simulink model "parrot_motor_speed"  (R2022a)
settings: Solver=FixedStepAuto  StartTime=0.0  StopTime=100  RelTol=1e-3  EnableMultiTasking=on
InitFcn:
  | load('BusDefinitions.mat')
undefined symbols (not defined in the file): codertarget, Ts
libraries: simulink x34
settings Model: SimulationMode=external  ExtModeTrigDuration=80  Creator=The MathWorks, Inc.  LastModifiedBy=Muhammad Ahmad Basra
settings SolverCC: AlgebraicLoopSolver=TrustRegion  PositivePriorityOrder=on
settings DataIOCC: ReturnWorkspaceOutputs=off
settings OptimizationCC: PassReuseOutputArgsThreshold=0  MaxStackSize=64
settings DebuggingCC: ParameterOverflowMsg=none  ParameterPrecisionLossMsg=none  ParameterTunabilityLossMsg=error  UnconnectedInputMsg=warning  UnconnectedOutputMsg=warning  UnconnectedLineMsg=warning  PregeneratedLibrarySubsystemCodeDiagnostic=none  SFMachineParentedDataDiag=warning  ArithmeticOperatorsInVariantConditions=warning
settings HardwareCC: ProdBitPerPointer=32  ProdBitPerSizeT=32  ProdBitPerPtrDiffT=32  ProdLargestAtomicInteger=Long  ProdWordSize=32  ProdHWDeviceType=ARM Compatible->ARM 9  UseEmbeddedCoderFeatures=off  UseSimulinkCoderFeatures=off
settings SFSimCC: SimUseLocalCustomCode=off  MATLABDynamicMemAlloc=off  CustomCodeUndefinedFunction=UseInterfaceOnly
settings RTWCC: SystemTargetFile=ert.tlc  HardwareBoard=PARROT Mambo  TemplateMakefile=ert_default_tmf  GenerateReport=on  RTWUseLocalCustomCode=off  Toolchain=Sourcery G++ Lite GNU Toolchain for Drones  LaunchReport=on
settings CodeAppCC: ForceParamTrailComments=on  OperatorAnnotations=on  StateflowObjectComments=on
settings ERTTargetCC: ERTCustomFileBanners=off  SupportContinuousTime=on  SupportNonInlinedSFcns=on  RemoveResetFunc=off  ModelStepFunctionPrototypeControlCompliant=off

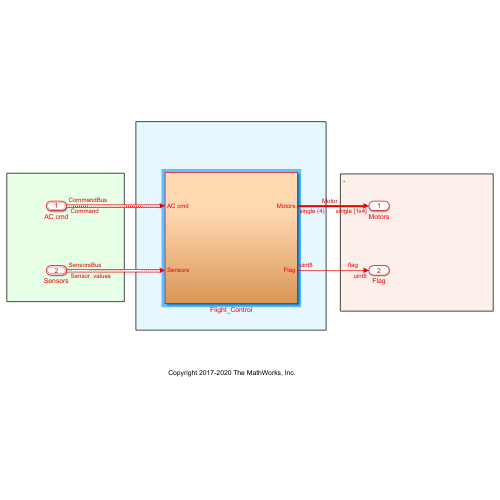
[thumbnail: Simulink's stored preview of the top-level diagram]
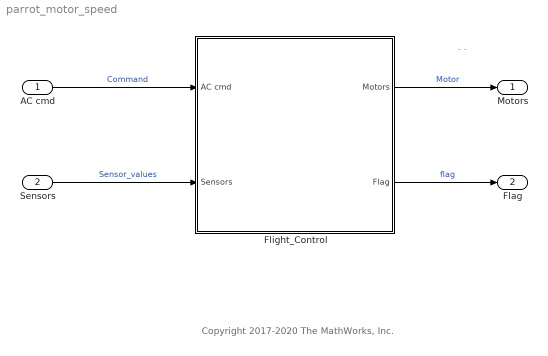
== system parrot_motor_speed ==
  note: .
      |
      |
      | .
  note: Copyright 2017-2020 The MathWorks, Inc.
  AC cmd : Inport  OutDataTypeStr=Bus: CommandBus  BusOutputAsStruct=on
  Sensors : Inport  Port=2  OutDataTypeStr=Bus: SensorsBus  BusOutputAsStruct=on
  Flight_Control : Subsystem  InitFcn=codertarget.parrot.internal.fcsSubsystemCallback(gcb);
  Motors : Outport  OutDataTypeStr=single  PortDimensions=[1 4]  VectorParamsAs1DForOutWhenUnconnected=off
  Flag : Outport  Port=2  OutDataTypeStr=uint8  PortDimensions=1  VectorParamsAs1DForOutWhenUnconnected=off
  wires:
  Flight_Control/1(Motors) -> Motors/1  "Motor"
  AC cmd/1 -> Flight_Control/1(AC cmd)  "Command"
  Sensors/1 -> Flight_Control/2(Sensors)  "Sensor_values"
  Flight_Control/2(Flag) -> Flag/1  "flag"

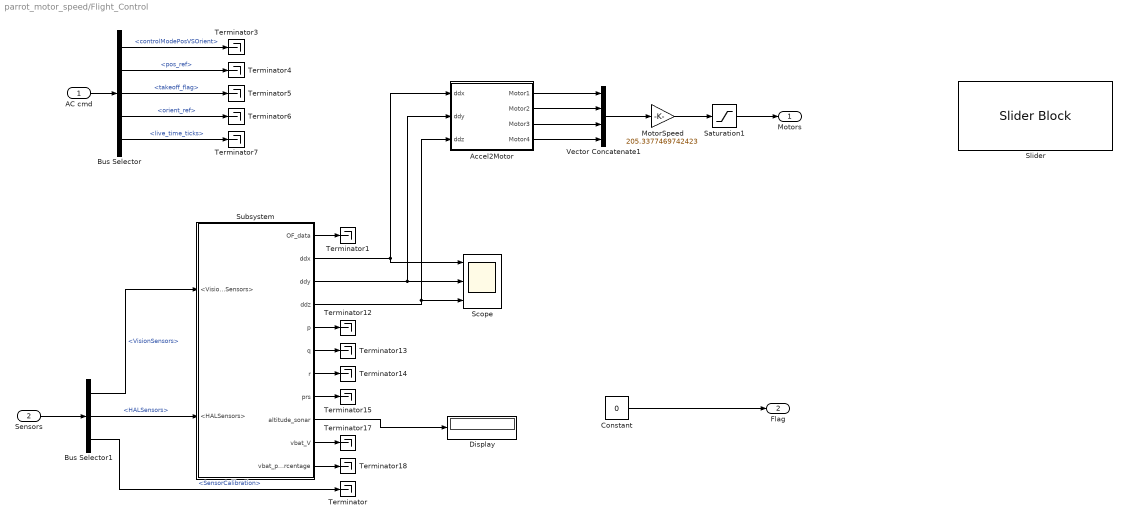
== system parrot_motor_speed/Flight_Control ==
  AC cmd : Inport
  Sensors : Inport  Port=2
  Accel2Motor : Subsystem
  Bus Selector : BusSelector  OutputSignals=controlModePosVSOrient,pos_ref,takeoff_flag,orient_ref,live_time_ticks
  Bus Selector1 : BusSelector  OutputSignals=VisionSensors,HALSensors,SensorCalibration
  Constant : Constant  Value=0  OutDataTypeStr=uint8  SampleTime=Ts
  Display : Display
  MotorSpeed : Gain  Gain=205.3377469742423  OutDataTypeStr=single
  Saturation1 : Saturate  UpperLimit=500  LowerLimit=0  OutDataTypeStr=single
  Scope : Scope  NumInputPorts=3
  Slider : SliderBlock  ScaleMax=500
  Subsystem : Subsystem
  Terminator{,1,3..7,12..15,17..18} (13 alike) : Terminator
  Vector Concatenate1 : Concatenate  NumInputs=4
  Motors : Outport  VectorParamsAs1DForOutWhenUnconnected=off
  Flag : Outport  Port=2  VectorParamsAs1DForOutWhenUnconnected=off
  wires:
  AC cmd/1 -> Bus Selector/1
  Sensors/1 -> Bus Selector1/1
  Bus Selector/1 -> Terminator3/1  "<controlModePosVSOrient>"
  Bus Selector/2 -> Terminator4/1  "<pos_ref>"
  Bus Selector/3 -> Terminator5/1  "<takeoff_flag>"
  Bus Selector/4 -> Terminator6/1  "<orient_ref>"
  Bus Selector/5 -> Terminator7/1  "<live_time_ticks>"
  Constant/1 -> Flag/1
  Vector Concatenate1/1 -> MotorSpeed/1
  Accel2Motor/1(Motor1) -> Vector Concatenate1/1
  Accel2Motor/4(Motor4) -> Vector Concatenate1/4
  Accel2Motor/2(Motor2) -> Vector Concatenate1/2
  Accel2Motor/3(Motor3) -> Vector Concatenate1/3
  Saturation1/1 -> Motors/1
  Bus Selector1/1 -> Subsystem/1(<VisionSensors>)  "<VisionSensors>"
  Bus Selector1/2 -> Subsystem/2(<HALSensors>)  "<HALSensors>"
  Bus Selector1/3 -> Terminator/1  "<SensorCalibration>"
  Subsystem/1(OF_data) -> Terminator1/1
  Subsystem/2(ddx) -> Accel2Motor/1(ddx), Scope/1
  Subsystem/3(ddy) -> Accel2Motor/2(ddy), Scope/2
  Subsystem/4(ddz) -> Accel2Motor/3(ddz), Scope/3
  Subsystem/5(p) -> Terminator12/1
  Subsystem/7(r) -> Terminator14/1
  Subsystem/8(prs) -> Terminator15/1
  Subsystem/9(altitude_sonar) -> Display/1
  Subsystem/10(vbat_V) -> Terminator17/1
  Subsystem/11(vbat_percentage) -> Terminator18/1
  Subsystem/6(q) -> Terminator13/1
  MotorSpeed/1 -> Saturation1/1

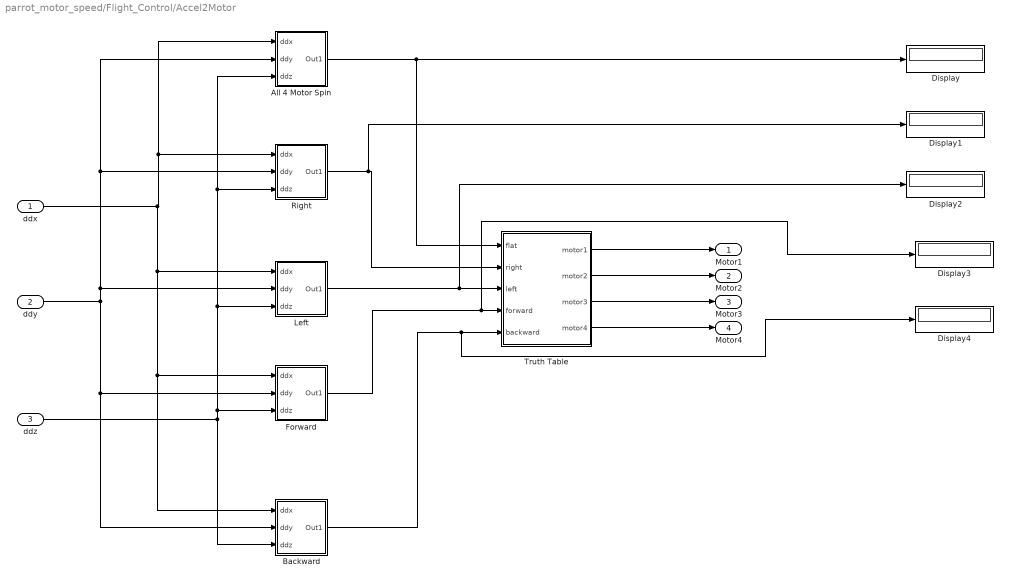
== system parrot_motor_speed/Flight_Control/Accel2Motor ==
  ddx : Inport
  ddy : Inport  Port=2
  ddz : Inport  Port=3
  All 4 Motor Spin : Subsystem
  Backward : Subsystem
  Display{,1..4} (5 alike) : Display
  Forward : Subsystem
  Left : Subsystem
  Right : Subsystem
  Truth Table : Truth Table  TreatAsAtomicUnit=on
  Motor1 : Outport  VectorParamsAs1DForOutWhenUnconnected=off
  Motor2 : Outport  Port=2  VectorParamsAs1DForOutWhenUnconnected=off
  Motor3 : Outport  Port=3  VectorParamsAs1DForOutWhenUnconnected=off
  Motor4 : Outport  Port=4  VectorParamsAs1DForOutWhenUnconnected=off
  wires:
  All 4 Motor Spin/1(Out1) -> Display/1, Truth Table/1(flat)
  Right/1(Out1) -> Display1/1, Truth Table/2(right)
  Left/1(Out1) -> Display2/1, Truth Table/3(left)
  Forward/1(Out1) -> Display3/1, Truth Table/4(forward)
  Backward/1(Out1) -> Display4/1, Truth Table/5(backward)
  Truth Table/1(motor1) -> Motor1/1
  Truth Table/2(motor2) -> Motor2/1
  Truth Table/3(motor3) -> Motor3/1
  Truth Table/4(motor4) -> Motor4/1
  ddx/1 -> Backward/1(ddx), Forward/1(ddx), Left/1(ddx), Right/1(ddx), All 4 Motor Spin/1(ddx)
  ddy/1 -> Left/2(ddy), Right/2(ddy), All 4 Motor Spin/2(ddy), Backward/2(ddy), Forward/2(ddy)
  ddz/1 -> Backward/3(ddz), All 4 Motor Spin/3(ddz), Right/3(ddz), Left/3(ddz), Forward/3(ddz)

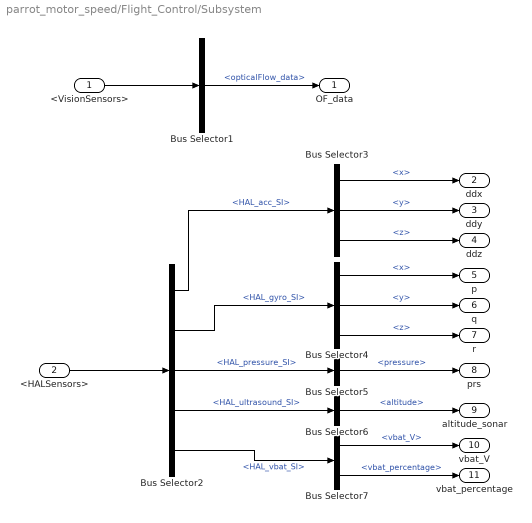
== system parrot_motor_speed/Flight_Control/Subsystem ==
  <VisionSensors> : Inport
  <HALSensors> : Inport  Port=2
  Bus Selector1 : BusSelector  OutputSignals=opticalFlow_data
  Bus Selector2 : BusSelector  OutputSignals=HAL_acc_SI,HAL_gyro_SI,HAL_pressure_SI,HAL_ultrasound_SI,HAL_vbat_SI
  Bus Selector3 : BusSelector  OutputSignals=x,y,z
  Bus Selector4 : BusSelector  OutputSignals=x,y,z
  Bus Selector5 : BusSelector  OutputSignals=pressure
  Bus Selector6 : BusSelector  OutputSignals=altitude
  Bus Selector7 : BusSelector  OutputSignals=vbat_V,vbat_percentage
  OF_data : Outport  VectorParamsAs1DForOutWhenUnconnected=off
  ddx : Outport  Port=2  VectorParamsAs1DForOutWhenUnconnected=off
  ddy : Outport  Port=3  VectorParamsAs1DForOutWhenUnconnected=off
  ddz : Outport  Port=4  VectorParamsAs1DForOutWhenUnconnected=off
  p : Outport  Port=5  VectorParamsAs1DForOutWhenUnconnected=off
  q : Outport  Port=6  VectorParamsAs1DForOutWhenUnconnected=off
  r : Outport  Port=7  VectorParamsAs1DForOutWhenUnconnected=off
  prs : Outport  Port=8  VectorParamsAs1DForOutWhenUnconnected=off
  altitude_sonar : Outport  Port=9  VectorParamsAs1DForOutWhenUnconnected=off
  vbat_V : Outport  Port=10  VectorParamsAs1DForOutWhenUnconnected=off
  vbat_percentage : Outport  Port=11  VectorParamsAs1DForOutWhenUnconnected=off
  wires:
  <VisionSensors>/1 -> Bus Selector1/1
  <HALSensors>/1 -> Bus Selector2/1
  Bus Selector1/1 -> OF_data/1  "<opticalFlow_data>"
  Bus Selector2/1 -> Bus Selector3/1  "<HAL_acc_SI>"
  Bus Selector2/2 -> Bus Selector4/1  "<HAL_gyro_SI>"
  Bus Selector2/3 -> Bus Selector5/1  "<HAL_pressure_SI>"
  Bus Selector2/4 -> Bus Selector6/1  "<HAL_ultrasound_SI>"
  Bus Selector2/5 -> Bus Selector7/1  "<HAL_vbat_SI>"
  Bus Selector3/1 -> ddx/1  "<x>"
  Bus Selector3/2 -> ddy/1  "<y>"
  Bus Selector3/3 -> ddz/1  "<z>"
  Bus Selector4/2 -> q/1  "<y>"
  Bus Selector4/1 -> p/1  "<x>"
  Bus Selector4/3 -> r/1  "<z>"
  Bus Selector5/1 -> prs/1  "<pressure>"
  Bus Selector6/1 -> altitude_sonar/1  "<altitude>"
  Bus Selector7/1 -> vbat_V/1  "<vbat_V>"
  Bus Selector7/2 -> vbat_percentage/1  "<vbat_percentage>"

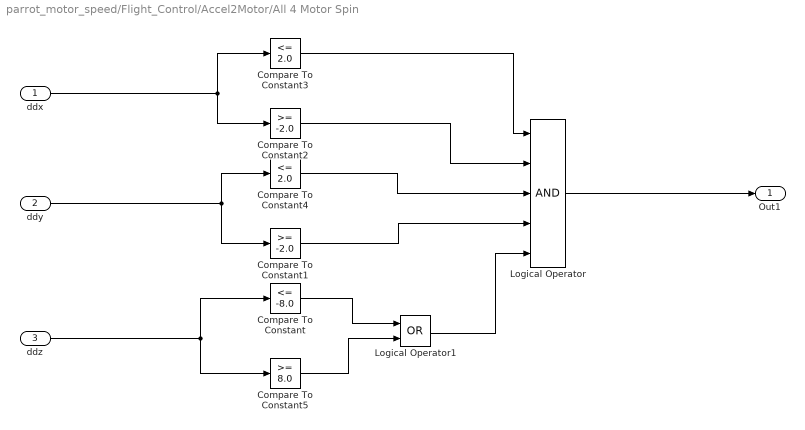
== system parrot_motor_speed/Flight_Control/Accel2Motor/All 4 Motor Spin ==
  ddx : Inport
  ddy : Inport  Port=2
  ddz : Inport  Port=3
  Compare To Constant : simulink/Logic and Bit Operations/Compare To Constant  relop=<=  const=-8.0  OutDataTypeStr=boolean
  Compare To Constant1 : simulink/Logic and Bit Operations/Compare To Constant  relop=>=  const=-2.0  OutDataTypeStr=boolean
  Compare To Constant2 : simulink/Logic and Bit Operations/Compare To Constant  relop=>=  const=-2.0  OutDataTypeStr=boolean
  Compare To Constant3 : simulink/Logic and Bit Operations/Compare To Constant  relop=<=  const=2.0  OutDataTypeStr=boolean
  Compare To Constant4 : simulink/Logic and Bit Operations/Compare To Constant  relop=<=  const=2.0  OutDataTypeStr=boolean
  Compare To Constant5 : simulink/Logic and Bit Operations/Compare To Constant  relop=>=  const=8.0  OutDataTypeStr=boolean
  Logical Operator : Logic  Inputs=5  AllPortsSameDT=off  OutDataTypeStr=boolean
  Logical Operator1 : Logic  Operator=OR  AllPortsSameDT=off  OutDataTypeStr=boolean
  Out1 : Outport  VectorParamsAs1DForOutWhenUnconnected=off
  wires:
  Compare To Constant4/1 -> Logical Operator/3
  ddy/1 -> Compare To Constant1/1, Compare To Constant4/1
  ddz/1 -> Compare To Constant5/1, Compare To Constant/1
  Compare To Constant/1 -> Logical Operator1/1
  ddx/1 -> Compare To Constant3/1, Compare To Constant2/1
  Compare To Constant1/1 -> Logical Operator/4
  Compare To Constant3/1 -> Logical Operator/1
  Logical Operator1/1 -> Logical Operator/5
  Compare To Constant5/1 -> Logical Operator1/2
  Compare To Constant2/1 -> Logical Operator/2
  Logical Operator/1 -> Out1/1

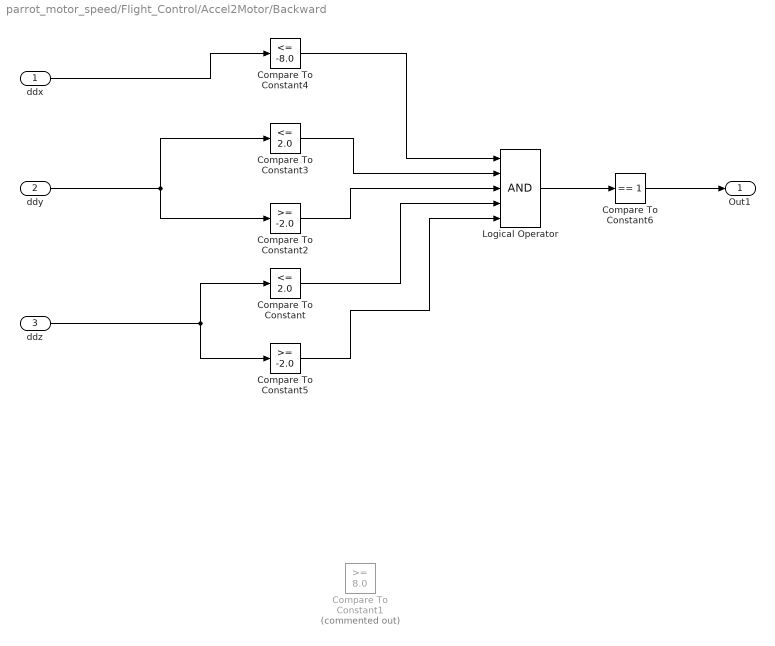
== system parrot_motor_speed/Flight_Control/Accel2Motor/Backward ==
  ddx : Inport
  ddy : Inport  Port=2
  ddz : Inport  Port=3
  Compare To Constant : simulink/Logic and Bit Operations/Compare To Constant  relop=<=  const=2.0  OutDataTypeStr=boolean
  Compare To Constant1 : simulink/Logic and Bit Operations/Compare To Constant  Commented=on  relop=>=  const=8.0  OutDataTypeStr=boolean
  Compare To Constant2 : simulink/Logic and Bit Operations/Compare To Constant  relop=>=  const=-2.0  OutDataTypeStr=boolean
  Compare To Constant3 : simulink/Logic and Bit Operations/Compare To Constant  relop=<=  const=2.0  OutDataTypeStr=boolean
  Compare To Constant4 : simulink/Logic and Bit Operations/Compare To Constant  relop=<=  const=-8.0  OutDataTypeStr=boolean
  Compare To Constant5 : simulink/Logic and Bit Operations/Compare To Constant  relop=>=  const=-2.0  OutDataTypeStr=boolean
  Compare To Constant6 : simulink/Logic and Bit Operations/Compare To Constant  relop===  const=1  OutDataTypeStr=boolean
  Logical Operator : Logic  Inputs=5  AllPortsSameDT=off  OutDataTypeStr=boolean
  Out1 : Outport  VectorParamsAs1DForOutWhenUnconnected=off
  wires:
  Compare To Constant2/1 -> Logical Operator/3
  Compare To Constant3/1 -> Logical Operator/2
  Compare To Constant4/1 -> Logical Operator/1
  ddx/1 -> Compare To Constant4/1
  ddy/1 -> Compare To Constant2/1, Compare To Constant3/1
  Compare To Constant6/1 -> Out1/1
  Logical Operator/1 -> Compare To Constant6/1
  Compare To Constant5/1 -> Logical Operator/5
  Compare To Constant/1 -> Logical Operator/4
  ddz/1 -> Compare To Constant5/1, Compare To Constant/1

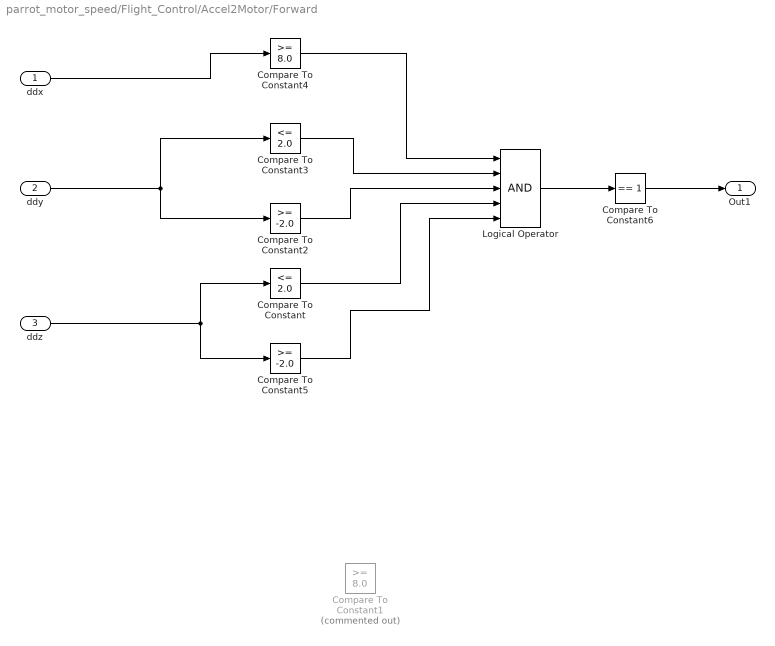
== system parrot_motor_speed/Flight_Control/Accel2Motor/Forward ==
  ddx : Inport
  ddy : Inport  Port=2
  ddz : Inport  Port=3
  Compare To Constant : simulink/Logic and Bit Operations/Compare To Constant  relop=<=  const=2.0  OutDataTypeStr=boolean
  Compare To Constant1 : simulink/Logic and Bit Operations/Compare To Constant  Commented=on  relop=>=  const=8.0  OutDataTypeStr=boolean
  Compare To Constant2 : simulink/Logic and Bit Operations/Compare To Constant  relop=>=  const=-2.0  OutDataTypeStr=boolean
  Compare To Constant3 : simulink/Logic and Bit Operations/Compare To Constant  relop=<=  const=2.0  OutDataTypeStr=boolean
  Compare To Constant4 : simulink/Logic and Bit Operations/Compare To Constant  relop=>=  const=8.0  OutDataTypeStr=boolean
  Compare To Constant5 : simulink/Logic and Bit Operations/Compare To Constant  relop=>=  const=-2.0  OutDataTypeStr=boolean
  Compare To Constant6 : simulink/Logic and Bit Operations/Compare To Constant  relop===  const=1  OutDataTypeStr=boolean
  Logical Operator : Logic  Inputs=5  AllPortsSameDT=off  OutDataTypeStr=boolean
  Out1 : Outport  VectorParamsAs1DForOutWhenUnconnected=off
  wires:
  ddz/1 -> Compare To Constant/1, Compare To Constant5/1
  Compare To Constant/1 -> Logical Operator/4
  Compare To Constant5/1 -> Logical Operator/5
  Logical Operator/1 -> Compare To Constant6/1
  Compare To Constant6/1 -> Out1/1
  ddy/1 -> Compare To Constant3/1, Compare To Constant2/1
  ddx/1 -> Compare To Constant4/1
  Compare To Constant4/1 -> Logical Operator/1
  Compare To Constant3/1 -> Logical Operator/2
  Compare To Constant2/1 -> Logical Operator/3

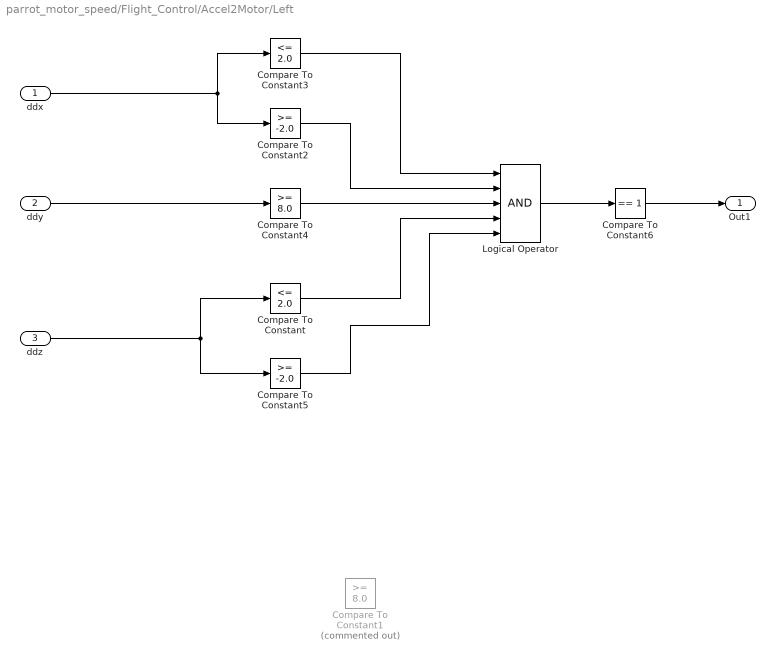
== system parrot_motor_speed/Flight_Control/Accel2Motor/Left ==
  ddx : Inport
  ddy : Inport  Port=2
  ddz : Inport  Port=3
  Compare To Constant : simulink/Logic and Bit Operations/Compare To Constant  relop=<=  const=2.0  OutDataTypeStr=boolean
  Compare To Constant1 : simulink/Logic and Bit Operations/Compare To Constant  Commented=on  relop=>=  const=8.0  OutDataTypeStr=boolean
  Compare To Constant2 : simulink/Logic and Bit Operations/Compare To Constant  relop=>=  const=-2.0  OutDataTypeStr=boolean
  Compare To Constant3 : simulink/Logic and Bit Operations/Compare To Constant  relop=<=  const=2.0  OutDataTypeStr=boolean
  Compare To Constant4 : simulink/Logic and Bit Operations/Compare To Constant  relop=>=  const=8.0  OutDataTypeStr=boolean
  Compare To Constant5 : simulink/Logic and Bit Operations/Compare To Constant  relop=>=  const=-2.0  OutDataTypeStr=boolean
  Compare To Constant6 : simulink/Logic and Bit Operations/Compare To Constant  relop===  const=1  OutDataTypeStr=boolean
  Logical Operator : Logic  Inputs=5  AllPortsSameDT=off  OutDataTypeStr=boolean
  Out1 : Outport  VectorParamsAs1DForOutWhenUnconnected=off
  wires:
  Compare To Constant6/1 -> Out1/1
  Logical Operator/1 -> Compare To Constant6/1
  Compare To Constant5/1 -> Logical Operator/5
  Compare To Constant/1 -> Logical Operator/4
  Compare To Constant4/1 -> Logical Operator/3
  Compare To Constant2/1 -> Logical Operator/2
  Compare To Constant3/1 -> Logical Operator/1
  ddy/1 -> Compare To Constant4/1
  ddz/1 -> Compare To Constant5/1, Compare To Constant/1
  ddx/1 -> Compare To Constant3/1, Compare To Constant2/1

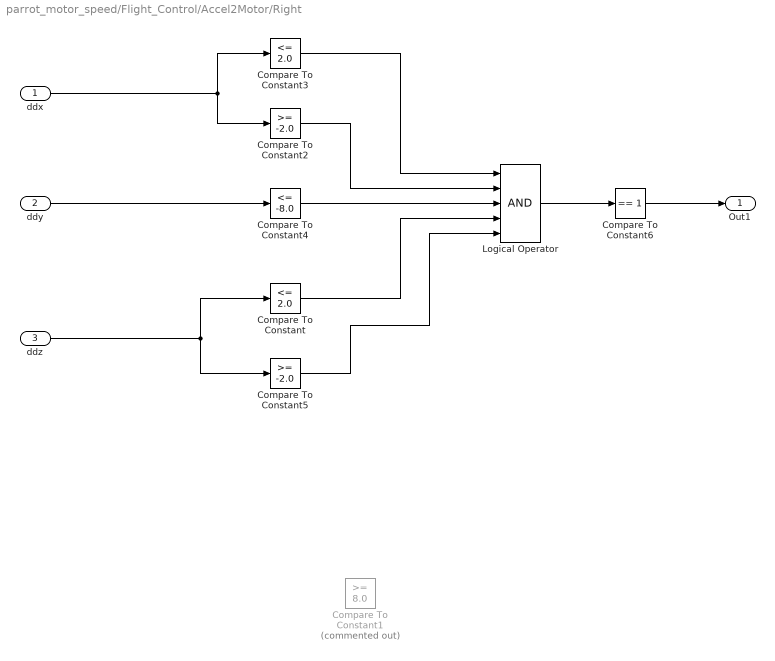
== system parrot_motor_speed/Flight_Control/Accel2Motor/Right ==
  ddx : Inport
  ddy : Inport  Port=2
  ddz : Inport  Port=3
  Compare To Constant : simulink/Logic and Bit Operations/Compare To Constant  relop=<=  const=2.0  OutDataTypeStr=boolean
  Compare To Constant1 : simulink/Logic and Bit Operations/Compare To Constant  Commented=on  relop=>=  const=8.0  OutDataTypeStr=boolean
  Compare To Constant2 : simulink/Logic and Bit Operations/Compare To Constant  relop=>=  const=-2.0  OutDataTypeStr=boolean
  Compare To Constant3 : simulink/Logic and Bit Operations/Compare To Constant  relop=<=  const=2.0  OutDataTypeStr=boolean
  Compare To Constant4 : simulink/Logic and Bit Operations/Compare To Constant  relop=<=  const=-8.0  OutDataTypeStr=boolean
  Compare To Constant5 : simulink/Logic and Bit Operations/Compare To Constant  relop=>=  const=-2.0  OutDataTypeStr=boolean
  Compare To Constant6 : simulink/Logic and Bit Operations/Compare To Constant  relop===  const=1  OutDataTypeStr=boolean
  Logical Operator : Logic  Inputs=5  AllPortsSameDT=off  OutDataTypeStr=boolean
  Out1 : Outport  VectorParamsAs1DForOutWhenUnconnected=off
  wires:
  ddx/1 -> Compare To Constant2/1, Compare To Constant3/1
  ddz/1 -> Compare To Constant/1, Compare To Constant5/1
  ddy/1 -> Compare To Constant4/1
  Compare To Constant3/1 -> Logical Operator/1
  Compare To Constant2/1 -> Logical Operator/2
  Compare To Constant4/1 -> Logical Operator/3
  Compare To Constant/1 -> Logical Operator/4
  Compare To Constant5/1 -> Logical Operator/5
  Logical Operator/1 -> Compare To Constant6/1
  Compare To Constant6/1 -> Out1/1

== matlab function parrot_motor_speed/Flight_Control/Accel2Motor/Truth Table ==
  data: flat input boolean; motor1 output boolean; right input boolean; left input boolean; forward input boolean; backward input boolean; motor2 output boolean; motor3 output boolean; motor4 output boolean
function [motor1, motor2, motor3, motor4] = fcn(flat, right, left, forward, backward)

INIT();

aVarTruthTableCondition_1 = false;
aVarTruthTableCondition_2 = false;
aVarTruthTableCondition_3 = false;
aVarTruthTableCondition_4 = false;
aVarTruthTableCondition_5 = false;


% Flat (UP/Down)

aVarTruthTableCondition_1 = logical(flat == 1);

% Right Bend

aVarTruthTableCondition_2 = logical(right == 1);

% Left Bend

aVarTruthTableCondition_3 = logical(left == 1);

% Forward Bend

aVarTruthTableCondition_4 = logical(forward == 1);

% backward Bend

aVarTruthTableCondition_5 = logical(backward == 1);

if (aVarTruthTableCondition_1 && ~aVarTruthTableCondition_2 && ~aVarTruthTableCondition_3 && ~aVarTruthTableCondition_4 && ~aVarTruthTableCondition_5)
    A1();
elseif (~aVarTruthTableCondition_1 && aVarTruthTableCondition_2 && ~aVarTruthTableCondition_3 && ~aVarTruthTableCondition_4 && ~aVarTruthTableCondition_5)
    A2();
elseif (~aVarTruthTableCondition_1 && ~aVarTruthTableCondition_2 && aVarTruthTableCondition_3 && ~aVarTruthTableCondition_4 && ~aVarTruthTableCondition_5)
    A3();
elseif (~aVarTruthTableCondition_1 && ~aVarTruthTableCondition_2 && ~aVarTruthTableCondition_3 && aVarTruthTableCondition_4 && ~aVarTruthTableCondition_5)
    A4();
elseif (~aVarTruthTableCondition_1 && ~aVarTruthTableCondition_2 && ~aVarTruthTableCondition_3 && ~aVarTruthTableCondition_4 && aVarTruthTableCondition_5)
    A5();
else % Default
    A6();
end

function INIT()

% Initial Action

coder.extrinsic('disp');
disp('truth table entered');
motor1=logical(0);
motor2=logical(0);
motor3=logical(0);
motor4=logical(0);

function A1()

% Spin all 4 Motors

motor1=logical(1);
motor2=logical(1);
motor3=logical(1);
motor4=logical(1);

function A2()

% Spin Motor 1 only

motor1=logical(1);

function A3()

% Spin Motor 2 only

motor2=logical(1);

function A4()

% Spin Motor 3 only

motor3=logical(1);

function A5()

% Spin Motor 4 only

motor4=logical(1);

function A6()

% Do not spin any motors

motor1=logical(0);
motor2=logical(0);
motor3=logical(0);
motor4=logical(0);
